simulink model "SprintDamper"  (R2021a)
settings: Solver=VariableStepAuto  StartTime=0.0  StopTime=10.0  RelTol=1e-3
settings Model: Creator=shreyas  LastModifiedBy=shreyas

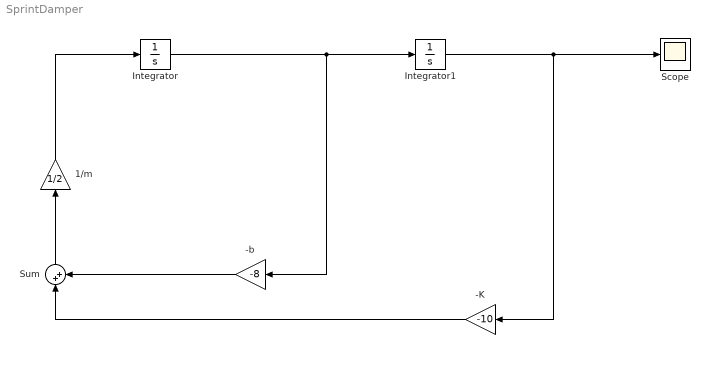
== system SprintDamper ==
  -K : Gain  Gain=-10
  -b : Gain  Gain=-8
  1/m : Gain  Gain=1/2
  "Integrator " : Integrator
  "Integrator1 " : Integrator  InitialCondition=1
  "Scope " : Scope
  Sum : Sum  Inputs=|++
  wires:
  1/m/1 -> "Integrator "/1
  -b/1 -> Sum/2
  Sum/1 -> 1/m/1
  "Integrator "/1 -> -b/1, "Integrator1 "/1
  -K/1 -> Sum/1
  "Integrator1 "/1 -> -K/1, "Scope "/1
